simulink model "a1animation"  (Simulink 8.1)
settings: Solver=ode45  StartTime=0.0  StopTime=1000  RelTol=1e-3
undefined symbols (not defined in the file or in its folder): drawAircraft
libraries: simulink x6
settings Model: Creator=beard  LastModifiedBy=asus
settings OptimizationCC: InitFltsAndDblsToZero=on
settings DebuggingCC: StrictBusMsg=Warning

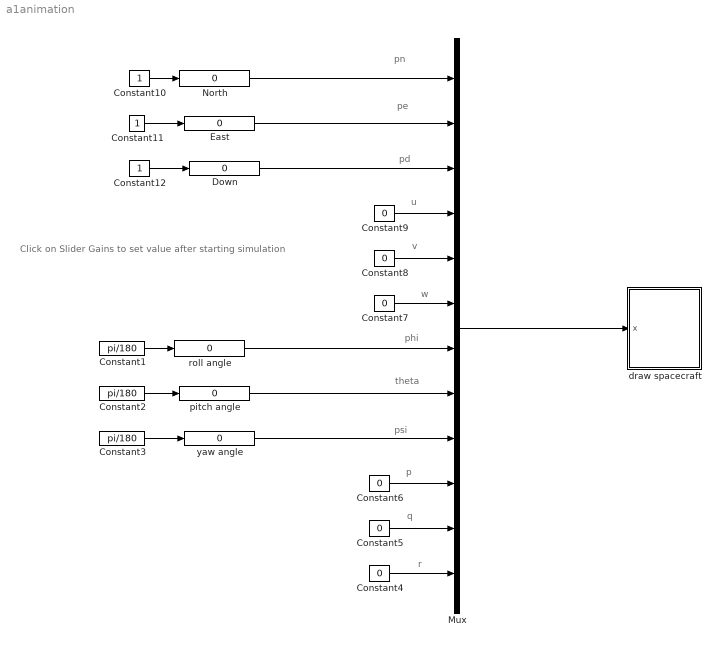
== system a1animation ==
  note: pn
  note: pe
  note: pd
  note: phi
  note: theta
  note: psi
  note: p
  note: q
  note: r
  note: u
  note: v
  note: w
  note: Click on Slider Gains to set value
      | after starting simulation
  Constant1 : Constant  Value=pi/180
  Constant10 : Constant
  Constant11 : Constant
  Constant12 : Constant
  Constant2 : Constant  Value=pi/180
  Constant3 : Constant  Value=pi/180
  Constant{4..9} (6 alike) : Constant  Value=0
  Down : simulink/Math Operations/Slider Gain  low=-10  gain=0  high=10
  East : simulink/Math Operations/Slider Gain  low=-10  gain=0  high=10
  Mux : Mux  Inputs=12
  North : simulink/Math Operations/Slider Gain  low=-10  gain=0  high=10
  draw spacecraft : Subsystem
      mask init:
      | % Define the vertices (physical location of vertices
      | %% MAV Dimention
      | ww=1;tww=0.5;fw=0.1;fl1=.3;fl2=0.2;
      | fl3=0.7;wl=0.25;twl=0.2;fh=0.2;th=-0.3;
      | 
      |   V = [...
      | 	 fl1       0          0;        ... % point 1
      |      fl2       0.5*fw     0.5*fh;   ... % point 2
      |      fl2      -0.5*fw     0.5*fh;   ... % point 3
      |      fl2      -0.5*fw    -0.5*fh;   ... % point 4
      | 	 fl2       0.5*fw    -0.5*fh;   ... % point 5
      |     -fl3       0          0;        ... % point 6
      |      0         0.5*ww     0;        ... % point 7
      |     -wl        0.5*ww     0;        ... % point 8
      | 	-wl       -0.5*ww     0;        ... % point 9
      |      0        -0.5*ww     0;        ... % point 10
      |     -fl3+twl   0.5*tww    0;        ... % point 11
      |     -fl3       0.5*tww    0;        ... % point 12
      |     -fl3      -0.5*tww    0;        ... % point 13
      |     -fl3+twl  -0.5*tww    0;        ... % point 14
      |     -fl3+twl   0          0;        ... % point 15
      |     -fl3       0          th;       ... % point 16
      |      fl1       0          0.05;     ... % point 17  near 1
      |     -fl3-0.05  0          0;        ... % point 18  near 6
      |   ];
      | 
      | % define faces as a list of vertices numbered above
      |   F = [...
      |       1, 2, 3, 1;...
      |       1, 3, 4, 1;...
      |       1, 4, 5, 1;...
      |       1, 5, 2, 1;...  % head
      |       
      |       2, 3, 6, 6;...
      |       3, 4, 6, 6;...
      |       4, 5, 6, 6;...
      |       5, 2, 6, 6;...  % body
      |       
      |       7, 8, 9, 10;...
      |       11, 12, 13, 14;... % wings
      |       
      |       6, 15, 16, 6;...
      |       
      |       
      |   
      |        % 1, 2,  6,  5;...  % front
      |        % 4, 3,  7,  8;...  % back
      |        % 1, 5,  8,  4;...  % right 
      |        % 2, 6,  7,  3;...  % left
      |        % 5, 6,  7,  8;...  % top
      |        % 9, 10, 11, 12;... % bottom
      |         ];
      | 
      | % define colors for each face    
      |   myred = [1, 0, 0];
      |   mygreen = [0, 1, 0];
      |   myblue = [0, 0, 1];
      |   myyellow = [1, 1, 0];
      |   mycyan = [0, 1, 1];
      | 
      |   patchcolors = [...
      |     myred;...    % front
      |     mygreen;...  % back
      |     myblue;...   % right
      |     myyellow;... % left
      |     mycyan;...   % top
      |     mycyan;...   % bottom
      |     myred;...    % front
      |     mygreen;...  % back
      |     myblue;...   % right
      |     myyellow;... % left
      |     mycyan;...   % top
      |    
      |     ];
      mask Display: image(imread('tv.jpg'))
  pitch angle : simulink/Math Operations/Slider Gain  low=-180  gain=0  high=180
  roll angle : simulink/Math Operations/Slider Gain  low=-180  gain=0  high=180
  "yaw angle " : simulink/Math Operations/Slider Gain  low=-180  gain=0  high=180
  wires:
  Mux/1 -> draw spacecraft/1(x)
  roll angle/1 -> Mux/7
  Constant1/1 -> roll angle/1
  pitch angle/1 -> Mux/8
  Constant2/1 -> pitch angle/1
  "yaw angle "/1 -> Mux/9
  Constant3/1 -> "yaw angle "/1
  Constant4/1 -> Mux/12
  Constant5/1 -> Mux/11
  Constant6/1 -> Mux/10
  Constant7/1 -> Mux/6
  Constant8/1 -> Mux/5
  Constant9/1 -> Mux/4
  North/1 -> Mux/1
  Constant10/1 -> North/1
  East/1 -> Mux/2
  Constant11/1 -> East/1
  Down/1 -> Mux/3
  Constant12/1 -> Down/1

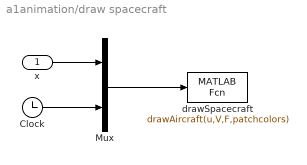
== system a1animation/draw spacecraft ==
  x : Inport
  Clock : Clock
  Mux : Mux  Inputs=2
  drawSpacecraft : MATLABFcn  MATLABFcn=drawAircraft(u,V,F,patchcolors)  OutputDimensions=0  SampleTime=0.1
  wires:
  Mux/1 -> drawSpacecraft/1
  x/1 -> Mux/1
  Clock/1 -> Mux/2
